simulink model "spwm_pmsm"  (R2020b)
settings: Solver=VariableStepAuto  StartTime=0.0  StopTime=2  FixedStep=1e-3  RelTol=1e-3
libraries: powerlib x9, simulink x3, powerlib_meascontrol x2
settings Model: Creator=matti  LastModifiedBy=matti

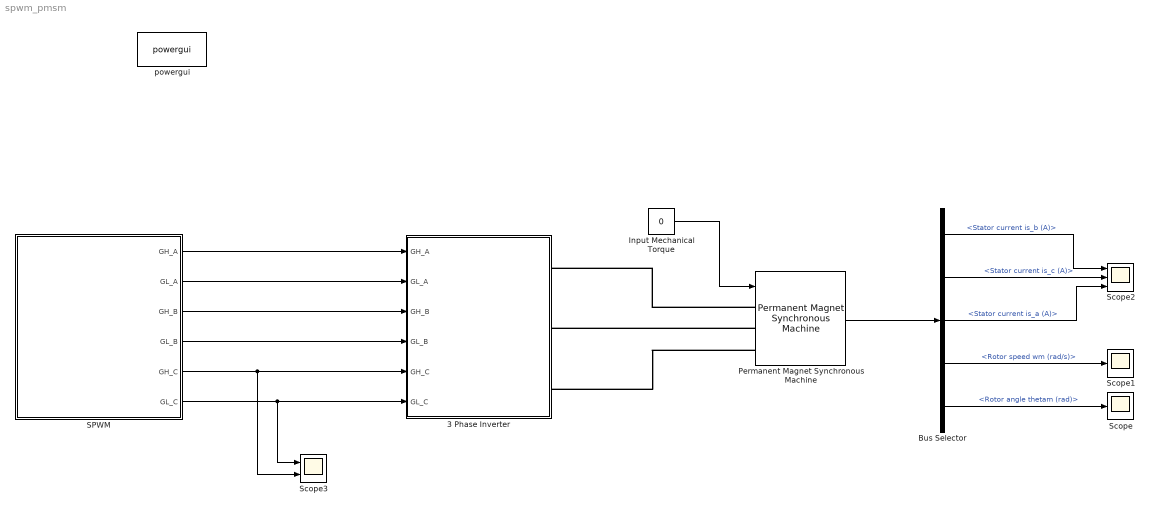
== system spwm_pmsm ==
  3 Phase Inverter : Subsystem
  Bus Selector : BusSelector  OutputSignals=Stator current is_b (A),Stator current is_c (A),Stator current is_a (A),Rotor speed wm (rad/s),Rotor angle thetam (rad)
  Input Mechanical Torque : Constant  Value=0
  Permanent Magnet Synchronous Machine : powerlib/Machines/Permanent Magnet Synchronous Machine  NbPhases=3  FluxDistribution=Sinusoidal  RotorType=Round  MechanicalLoad=Torque Tm  PresetModel=No  ShowDetailedParameters=on  MeasurementBus=off  Resistance=0.0485  Inductance=8.5e-3  dqInductances=[8.5e-3,8.5e-3]  La=0.000395  MachineConstant=Flux linkage established by magnets (V.s)  Flux=0.1194  VoltageCst=86.6271  TorqueCst=0.7164  Flat=120  Mechanical=[0.0027 0.0004924 4 0]  PolePairs=4  InitialConditions=[0,0, 0,0]  InitialConditions5ph=[0 0 0 0 0 0]  RefAngle=90 degrees behind phase A axis (modified Park)  IterativeDiscreteModel=Trapezoidal non iterative  TsBlock=-1  TsPowergui=0
  SPWM : Subsystem
  Scope : Scope
  Scope1 : Scope
  Scope2 : Scope  NumInputPorts=3
  Scope3 : Scope  NumInputPorts=2
  powergui : powerlib/powergui  Priority=1  SimulationMode=Continuous  SampleTime=50e-6  frequency=60  Iterations=50  frequencyindice=0  Pbase=100e6  ErrMax=1e-4  UnitsV=kV  UnitsW=MW  buscounter=0  FunctionMessages=off  echomessages=off  EnableUseOfTLC=off  CurrentSourceSwitches=off  DisableSnubberDevices=off  DisableRonSwitches=off  DisableVfSwitches=off  DisplayEquations=off  AutomaticDiscreteSolvers=off  SolverType=Tustin/Backward Euler (TBE)  Interpol=off  ExternalGateDelay=off  methode=off  Ts=100  x0status=blocks  SPID=on  SwTol=0  HookPort=off  NonlinearTolerance=1e-4  nMaxIteration=100  ContinueOnMaxIteration=off  RestoreLinks=warning  ResistiveCurrentMeasurement=off  Frange=[0:2:500]  Ylog=off  Xlog=on  ShowGrid=off  save=off  variable=ZData  structure=0  ZoomFFT=off  StartTime=0.0  cycles=1  DisplayStyle=1  fundamental=60  FreqAxis=off  MaxFrequency=1000  frequencyindicesteady=1  RmsSteady=1  display=off
  wires:
  Input Mechanical Torque/1 -> Permanent Magnet Synchronous Machine/1
  Permanent Magnet Synchronous Machine/1 -> Bus Selector/1
  Bus Selector/5 -> Scope/1  "<Rotor angle thetam (rad)>"
  Bus Selector/4 -> Scope1/1  "<Rotor speed wm (rad/s)>"
  Bus Selector/2 -> Scope2/2  "<Stator current is_c (A)>"
  Bus Selector/3 -> Scope2/3  "<Stator current is_a (A)>"
  SPWM/1(GH_A) -> 3 Phase Inverter/1(GH_A)
  SPWM/2(GL_A) -> 3 Phase Inverter/2(GL_A)
  SPWM/3(GH_B) -> 3 Phase Inverter/3(GH_B)
  SPWM/4(GL_B) -> 3 Phase Inverter/4(GL_B)
  SPWM/5(GH_C) -> Scope3/2, 3 Phase Inverter/5(GH_C)
  SPWM/6(GL_C) -> Scope3/1, 3 Phase Inverter/6(GL_C)
  Bus Selector/1 -> Scope2/1  "<Stator current is_b (A)>"
  connections:
  Permanent Magnet Synchronous Machine/LConn1 -- 3 Phase Inverter/RConn1
  Permanent Magnet Synchronous Machine/LConn2 -- 3 Phase Inverter/RConn2
  Permanent Magnet Synchronous Machine/LConn3 -- 3 Phase Inverter/RConn3

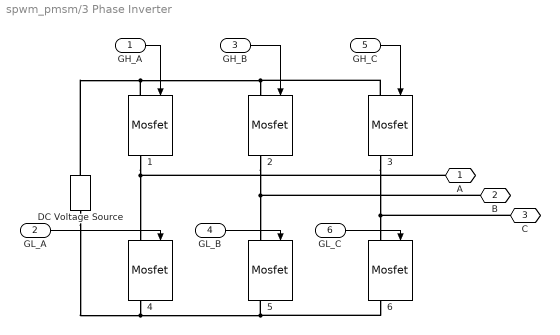
== system spwm_pmsm/3 Phase Inverter ==
  GH_A : Inport
  GL_A : Inport  Port=2
  GH_B : Inport  Port=3
  GL_B : Inport  Port=4
  GH_C : Inport  Port=5
  GL_C : Inport  Port=6
  {1..6} (6 alike) : powerlib/Power Electronics/Mosfet  Ron=0.1  Lon=0  Rd=0.01  Vfd=0  IC=0  Rs=1e5  Cs=inf  Measurements=on
  DC Voltage Source : powerlib/Electrical Sources/DC Voltage Source  Amplitude=100  Measurements=None
  A : PMIOPort  Side=Right
  B : PMIOPort  Port=2  Side=Right
  C : PMIOPort  Port=3  Side=Right
  wires:
  GH_C/1 -> 3/1
  GL_A/1 -> 4/1
  GH_B/1 -> 2/1
  GL_C/1 -> 6/1
  GL_B/1 -> 5/1
  GH_A/1 -> 1/1
  connections:
  4/RConn1 -- DC Voltage Source/LConn1 -- 6/RConn1 -- 5/RConn1
  2/RConn1 -- 5/LConn1 -- B/RConn1
  1/LConn1 -- DC Voltage Source/RConn1 -- 3/LConn1 -- 2/LConn1
  3/RConn1 -- C/RConn1 -- 6/LConn1
  1/RConn1 -- 4/LConn1 -- A/RConn1

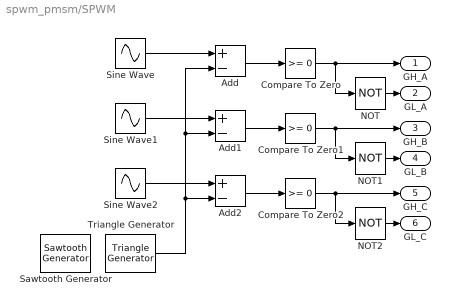
== system spwm_pmsm/SPWM ==
  Add : Sum  Inputs=+-
  Add1 : Sum  Inputs=+-
  Add2 : Sum  Inputs=+-
  Compare To Zero : simulink/Logic and Bit Operations/Compare To Zero  relop=>=  OutDataTypeStr=boolean
  Compare To Zero1 : simulink/Logic and Bit Operations/Compare To Zero  relop=>=  OutDataTypeStr=boolean
  Compare To Zero2 : simulink/Logic and Bit Operations/Compare To Zero  relop=>=  OutDataTypeStr=boolean
  NOT : Logic  Operator=NOT  IconShape=distinctive  AllPortsSameDT=off  OutDataTypeStr=boolean
  NOT1 : Logic  Operator=NOT  IconShape=distinctive  AllPortsSameDT=off  OutDataTypeStr=boolean
  NOT2 : Logic  Operator=NOT  IconShape=distinctive  AllPortsSameDT=off  OutDataTypeStr=boolean
  Sawtooth Generator : powerlib_meascontrol/Pulse & Signal Generators/Sawtooth Generator  Freq=1e4  Phase=180  Ts=0
  Sine Wave : Sin  Frequency=2*pi*50  SampleTime=0
  Sine Wave1 : Sin  Frequency=2*pi*50  Phase=2*pi/3  SampleTime=0
  Sine Wave2 : Sin  Frequency=2*pi*50  Phase=-2*pi/3  SampleTime=0
  Triangle Generator : powerlib_meascontrol/Pulse & Signal Generators/Triangle Generator  Freq=1e4  Phase=90  Ts=0
  GH_A : Outport
  GL_A : Outport  Port=2
  GH_B : Outport  Port=3
  GL_B : Outport  Port=4
  GH_C : Outport  Port=5
  GL_C : Outport  Port=6
  wires:
  Add1/1 -> Compare To Zero1/1
  Sine Wave1/1 -> Add1/1
  Sine Wave2/1 -> Add2/1
  Compare To Zero/1 -> GH_A/1, NOT/1
  Add/1 -> Compare To Zero/1
  Add2/1 -> Compare To Zero2/1
  Sine Wave/1 -> Add/1
  NOT/1 -> GL_A/1
  Compare To Zero1/1 -> GH_B/1, NOT1/1
  NOT1/1 -> GL_B/1
  Compare To Zero2/1 -> GH_C/1, NOT2/1
  NOT2/1 -> GL_C/1
  Triangle Generator/1 -> Add/2, Add1/2, Add2/2
